simulink model "Feeder_1"  (Simulink 8.8)
settings: Solver=ode4  StartTime=0.0  StopTime=inf  FixedStep=Ts  RelTol=1e-3  EnableMultiTasking=on
PreLoadFcn:
  | Ts=125e-6;Core_Num = 0; np=1; nq=1; Vmin=.9;
PostLoadFcn:
  | Ts=125e-6;Core_Num = 0; np=1; nq=1; Vmin=.9;
InitFcn:
  | Ts=125e-6;Core_Num = 0; np=1; nq=1; Vmin=.9;
undefined symbols (not defined in the file or in its folder): another_event_name, DiscIntNeverNeededParam, I, j, Left, my_event_name, Right, type, V, X
libraries: powerlib x316, powerlib_meascontrol x227, simulink_extras x78, simulink x25, rtio_generic_c37_118 x22, ssn_lib x9, rtlab x6, powerlib_extras x3, artemis x1, rtio_opalrt_ml605ex1 x1, rtio_spectracom x1, rtio_generic_ethernet x1
(part 8 of 14)

== system Feeder_1/SS_PMU/Subsystem42/Subsystem ==
  In1 : Inport
  Bus Creator : BusCreator  Inputs=3
  Selector1 : Selector  InputPortWidth=14  IndexOptions=Index vector (dialog)  Indices=[13]  OutputSizes=1
  Selector2 : Selector  InputPortWidth=14  IndexOptions=Index vector (dialog)  Indices=[14]  OutputSizes=1
  Selector5 : Selector  InputPortWidth=14  IndexOptions=Index vector (dialog)  Indices=[1 2 3 4 5 6 7 8 9 10 11 12]  OutputSizes=1
  Out1 : Outport
  wires:
  In1/1 -> Selector5/1, Selector2/1, Selector1/1
  Selector5/1 -> Bus Creator/1  "Measurements"
  Bus Creator/1 -> Out1/1
  Selector1/1 -> Bus Creator/2  "FREQ"
  Selector2/1 -> Bus Creator/3  "FROC"

== system Feeder_1/SS_PMU/Subsystem43/Subsystem ==
  In1 : Inport
  Bus Creator : BusCreator  Inputs=3
  Selector1 : Selector  InputPortWidth=14  IndexOptions=Index vector (dialog)  Indices=[13]  OutputSizes=1
  Selector2 : Selector  InputPortWidth=14  IndexOptions=Index vector (dialog)  Indices=[14]  OutputSizes=1
  Selector5 : Selector  InputPortWidth=14  IndexOptions=Index vector (dialog)  Indices=[1 2 3 4 5 6 7 8 9 10 11 12]  OutputSizes=1
  Out1 : Outport
  wires:
  In1/1 -> Selector5/1, Selector2/1, Selector1/1
  Selector5/1 -> Bus Creator/1  "Measurements"
  Bus Creator/1 -> Out1/1
  Selector1/1 -> Bus Creator/2  "FREQ"
  Selector2/1 -> Bus Creator/3  "FROC"

== system Feeder_1/SS_PMU/Subsystem44/Subsystem ==
  In1 : Inport
  Bus Creator : BusCreator  Inputs=3
  Selector1 : Selector  InputPortWidth=14  IndexOptions=Index vector (dialog)  Indices=[13]  OutputSizes=1
  Selector2 : Selector  InputPortWidth=14  IndexOptions=Index vector (dialog)  Indices=[14]  OutputSizes=1
  Selector5 : Selector  InputPortWidth=14  IndexOptions=Index vector (dialog)  Indices=[1 2 3 4 5 6 7 8 9 10 11 12]  OutputSizes=1
  Out1 : Outport
  wires:
  In1/1 -> Selector5/1, Selector2/1, Selector1/1
  Selector5/1 -> Bus Creator/1  "Measurements"
  Bus Creator/1 -> Out1/1
  Selector1/1 -> Bus Creator/2  "FREQ"
  Selector2/1 -> Bus Creator/3  "FROC"

== system Feeder_1/SS_PMU/Subsystem5/Subsystem ==
  Measurements1 : Inport
  Demux7 : Demux  Outputs=2
  Subsystem1 : Subsystem
  Phasors_Vabc : Outport
  Phasors_Iabc : Outport  Port=2
  Phasor_Freq : Outport  Port=3
  Phasor_DTFreq : Outport  Port=4
  wires:
  Measurements1/1 -> Subsystem1/1(Measurements)
  Subsystem1/2(Phasors_Freq) -> Phasor_Freq/1
  Subsystem1/3(Phasors_DTFreq) -> Phasor_DTFreq/1
  Demux7/2 -> Phasors_Iabc/1
  Demux7/1 -> Phasors_Vabc/1
  Subsystem1/1(Phasors_abc) -> Demux7/1

== system Feeder_1/SS_PMU/Subsystem6/Subsystem ==
  Measurements1 : Inport
  Demux7 : Demux  Outputs=2
  Subsystem1 : Subsystem
  Phasors_Vabc : Outport
  Phasors_Iabc : Outport  Port=2
  Phasor_Freq : Outport  Port=3
  Phasor_DTFreq : Outport  Port=4
  wires:
  Measurements1/1 -> Subsystem1/1(Measurements)
  Subsystem1/2(Phasors_Freq) -> Phasor_Freq/1
  Subsystem1/3(Phasors_DTFreq) -> Phasor_DTFreq/1
  Demux7/2 -> Phasors_Iabc/1
  Demux7/1 -> Phasors_Vabc/1
  Subsystem1/1(Phasors_abc) -> Demux7/1

== system Feeder_1/SS_PMU/Subsystem7/Subsystem ==
  Measurements1 : Inport
  Demux7 : Demux  Outputs=2
  Subsystem1 : Subsystem
  Phasors_Vabc : Outport
  Phasors_Iabc : Outport  Port=2
  Phasor_Freq : Outport  Port=3
  Phasor_DTFreq : Outport  Port=4
  wires:
  Measurements1/1 -> Subsystem1/1(Measurements)
  Subsystem1/2(Phasors_Freq) -> Phasor_Freq/1
  Subsystem1/3(Phasors_DTFreq) -> Phasor_DTFreq/1
  Demux7/2 -> Phasors_Iabc/1
  Demux7/1 -> Phasors_Vabc/1
  Subsystem1/1(Phasors_abc) -> Demux7/1

== system Feeder_1/SS_PMU/Subsystem8/Subsystem ==
  Measurements1 : Inport
  Demux7 : Demux  Outputs=2
  Subsystem1 : Subsystem
  Phasors_Vabc : Outport
  Phasors_Iabc : Outport  Port=2
  Phasor_Freq : Outport  Port=3
  Phasor_DTFreq : Outport  Port=4
  wires:
  Measurements1/1 -> Subsystem1/1(Measurements)
  Subsystem1/2(Phasors_Freq) -> Phasor_Freq/1
  Subsystem1/3(Phasors_DTFreq) -> Phasor_DTFreq/1
  Demux7/2 -> Phasors_Iabc/1
  Demux7/1 -> Phasors_Vabc/1
  Subsystem1/1(Phasors_abc) -> Demux7/1

== system Feeder_1/SS_PMU/Subsystem9/Subsystem ==
  Measurements1 : Inport
  Demux7 : Demux  Outputs=2
  Subsystem1 : Subsystem
  Phasors_Vabc : Outport
  Phasors_Iabc : Outport  Port=2
  Phasor_Freq : Outport  Port=3
  Phasor_DTFreq : Outport  Port=4
  wires:
  Measurements1/1 -> Subsystem1/1(Measurements)
  Subsystem1/2(Phasors_Freq) -> Phasor_Freq/1
  Subsystem1/3(Phasors_DTFreq) -> Phasor_DTFreq/1
  Demux7/2 -> Phasors_Iabc/1
  Demux7/1 -> Phasors_Vabc/1
  Subsystem1/1(Phasors_abc) -> Demux7/1

== system Feeder_1/SM_NG/Dynamic Load BCDC2/Single-Phase Dynamic Load1/model ==
  v : Inport
  PQ : Inport  Port=2
  Break  Alg. Loop1 : Subsystem
  Complex to Magnitude-Angle : ComplexToMagnitudeAngle
  Complex to Real-Imag1 : ComplexToRealImag
  Constant : Constant
  Demux : Demux  Outputs=2
  Divide : Product  Inputs=**
  Gain : Gain  Gain=1.0114
  IC1 : InitialCondition
  IC2 : InitialCondition
  Magnitude-Angle to Complex : MagnitudeAngleToComplex
  PLL : Subsystem  mask{freq=fnom}
      mask prompts: freq "Initial frequency (Hz)"
  Positive Sequence  current : Subsystem
  RMS1 : powerlib_meascontrol/Measurements/RMS  TrueRMS=on  Freq=fnom  RMSInit=1  Ts=0
  Real-Imag to Complex : RealImagToComplex
  Real-Imag to Complex1 : RealImagToComplex
  Sum : Sum
  Transfer Fcn1 : TransferFcn  Numerator=[1 290.1]  Denominator=[1 298.8]
  Trigonometric Function1 : Trigonometry
  V> pu : Gain  Gain=1/Vbase/sqrt(3)  SaturateOnIntegerOverflow=on  OutDataTypeStr=Inherit: Same as input  ParamDataTypeStr=Inherit: Same as input
  V> pu1 : Gain  Gain=sqrt(2)  SaturateOnIntegerOverflow=on  OutDataTypeStr=Inherit: Same as input  ParamDataTypeStr=Inherit: Same as input
  i : Outport
  wires:
  V> pu/1 -> PLL/1(v (pu)), V> pu1/1
  Real-Imag to Complex/1 -> Positive Sequence  current/1(V1(pu))
  PQ/1 -> Demux/1
  Demux/1 -> Real-Imag to Complex1/1
  Demux/2 -> Real-Imag to Complex1/2
  Real-Imag to Complex1/1 -> Positive Sequence  current/2(S_ext)
  Complex to Real-Imag1/1 -> Real-Imag to Complex/1
  Complex to Real-Imag1/2 -> Real-Imag to Complex/2
  Magnitude-Angle to Complex/1 -> Complex to Real-Imag1/1
  Constant/1 -> PLL/2(freq (pu))
  PLL/1(alpha (rad)) -> Magnitude-Angle to Complex/2
  Complex to Magnitude-Angle/2 -> Sum/2
  PLL/2(wt) -> Sum/1
  Sum/1 -> Trigonometric Function1/1
  Trigonometric Function1/1 -> Divide/2
  Complex to Magnitude-Angle/1 -> Divide/1
  RMS1/1 -> IC1/1
  V> pu1/1 -> RMS1/1
  v/1 -> IC2/1
  Positive Sequence  current/1(I1(A)) -> Break  Alg. Loop1/1(In)
  Break  Alg. Loop1/1(Out) -> Complex to Magnitude-Angle/1
  IC1/1 -> Magnitude-Angle to Complex/1
  IC2/1 -> V> pu/1
  Transfer Fcn1/1 -> Gain/1
  Gain/1 -> i/1
  Divide/1 -> Transfer Fcn1/1

== system Feeder_1/SM_NG/Dynamic Load BCDC2/Single-Phase Dynamic Load2/model ==
  v : Inport
  PQ : Inport  Port=2
  Break  Alg. Loop1 : Subsystem
  Complex to Magnitude-Angle : ComplexToMagnitudeAngle
  Complex to Real-Imag1 : ComplexToRealImag
  Constant : Constant
  Demux : Demux  Outputs=2
  Divide : Product  Inputs=**
  Gain : Gain  Gain=1.0114
  IC1 : InitialCondition
  IC2 : InitialCondition
  Magnitude-Angle to Complex : MagnitudeAngleToComplex
  PLL : Subsystem  mask{freq=fnom}
      mask prompts: freq "Initial frequency (Hz)"
  Positive Sequence  current : Subsystem
  RMS1 : powerlib_meascontrol/Measurements/RMS  TrueRMS=on  Freq=fnom  RMSInit=1  Ts=0
  Real-Imag to Complex : RealImagToComplex
  Real-Imag to Complex1 : RealImagToComplex
  Sum : Sum
  Transfer Fcn1 : TransferFcn  Numerator=[1 290.1]  Denominator=[1 298.8]
  Trigonometric Function1 : Trigonometry
  V> pu : Gain  Gain=1/Vbase/sqrt(3)  SaturateOnIntegerOverflow=on  OutDataTypeStr=Inherit: Same as input  ParamDataTypeStr=Inherit: Same as input
  V> pu1 : Gain  Gain=sqrt(2)  SaturateOnIntegerOverflow=on  OutDataTypeStr=Inherit: Same as input  ParamDataTypeStr=Inherit: Same as input
  i : Outport
  wires:
  V> pu/1 -> PLL/1(v (pu)), V> pu1/1
  Real-Imag to Complex/1 -> Positive Sequence  current/1(V1(pu))
  PQ/1 -> Demux/1
  Demux/1 -> Real-Imag to Complex1/1
  Demux/2 -> Real-Imag to Complex1/2
  Real-Imag to Complex1/1 -> Positive Sequence  current/2(S_ext)
  Complex to Real-Imag1/1 -> Real-Imag to Complex/1
  Complex to Real-Imag1/2 -> Real-Imag to Complex/2
  Magnitude-Angle to Complex/1 -> Complex to Real-Imag1/1
  Constant/1 -> PLL/2(freq (pu))
  PLL/1(alpha (rad)) -> Magnitude-Angle to Complex/2
  Complex to Magnitude-Angle/2 -> Sum/2
  PLL/2(wt) -> Sum/1
  Sum/1 -> Trigonometric Function1/1
  Trigonometric Function1/1 -> Divide/2
  Complex to Magnitude-Angle/1 -> Divide/1
  RMS1/1 -> IC1/1
  V> pu1/1 -> RMS1/1
  v/1 -> IC2/1
  Positive Sequence  current/1(I1(A)) -> Break  Alg. Loop1/1(In)
  Break  Alg. Loop1/1(Out) -> Complex to Magnitude-Angle/1
  IC1/1 -> Magnitude-Angle to Complex/1
  IC2/1 -> V> pu/1
  Transfer Fcn1/1 -> Gain/1
  Gain/1 -> i/1
  Divide/1 -> Transfer Fcn1/1

== system Feeder_1/SM_NG/Dynamic Load BCDC2/Single-Phase Dynamic Load9/model ==
  v : Inport
  PQ : Inport  Port=2
  Break  Alg. Loop1 : Subsystem
  Complex to Magnitude-Angle : ComplexToMagnitudeAngle
  Complex to Real-Imag1 : ComplexToRealImag
  Constant : Constant
  Demux : Demux  Outputs=2
  Divide : Product  Inputs=**
  Gain : Gain  Gain=1.0114
  IC1 : InitialCondition
  IC2 : InitialCondition
  Magnitude-Angle to Complex : MagnitudeAngleToComplex
  PLL : Subsystem  mask{freq=fnom}
      mask prompts: freq "Initial frequency (Hz)"
  Positive Sequence  current : Subsystem
  RMS1 : powerlib_meascontrol/Measurements/RMS  TrueRMS=on  Freq=fnom  RMSInit=1  Ts=0
  Real-Imag to Complex : RealImagToComplex
  Real-Imag to Complex1 : RealImagToComplex
  Sum : Sum
  Transfer Fcn1 : TransferFcn  Numerator=[1 290.1]  Denominator=[1 298.8]
  Trigonometric Function1 : Trigonometry
  V> pu : Gain  Gain=1/Vbase/sqrt(3)  SaturateOnIntegerOverflow=on  OutDataTypeStr=Inherit: Same as input  ParamDataTypeStr=Inherit: Same as input
  V> pu1 : Gain  Gain=sqrt(2)  SaturateOnIntegerOverflow=on  OutDataTypeStr=Inherit: Same as input  ParamDataTypeStr=Inherit: Same as input
  i : Outport
  wires:
  V> pu/1 -> PLL/1(v (pu)), V> pu1/1
  Real-Imag to Complex/1 -> Positive Sequence  current/1(V1(pu))
  PQ/1 -> Demux/1
  Demux/1 -> Real-Imag to Complex1/1
  Demux/2 -> Real-Imag to Complex1/2
  Real-Imag to Complex1/1 -> Positive Sequence  current/2(S_ext)
  Complex to Real-Imag1/1 -> Real-Imag to Complex/1
  Complex to Real-Imag1/2 -> Real-Imag to Complex/2
  Magnitude-Angle to Complex/1 -> Complex to Real-Imag1/1
  Constant/1 -> PLL/2(freq (pu))
  PLL/1(alpha (rad)) -> Magnitude-Angle to Complex/2
  Complex to Magnitude-Angle/2 -> Sum/2
  PLL/2(wt) -> Sum/1
  Sum/1 -> Trigonometric Function1/1
  Trigonometric Function1/1 -> Divide/2
  Complex to Magnitude-Angle/1 -> Divide/1
  RMS1/1 -> IC1/1
  V> pu1/1 -> RMS1/1
  v/1 -> IC2/1
  Positive Sequence  current/1(I1(A)) -> Break  Alg. Loop1/1(In)
  Break  Alg. Loop1/1(Out) -> Complex to Magnitude-Angle/1
  IC1/1 -> Magnitude-Angle to Complex/1
  IC2/1 -> V> pu/1
  Transfer Fcn1/1 -> Gain/1
  Gain/1 -> i/1
  Divide/1 -> Transfer Fcn1/1

== system Feeder_1/SM_NG/Dynamic Load BCDC3/Single-Phase Dynamic Load1/model ==
  v : Inport
  PQ : Inport  Port=2
  Break  Alg. Loop1 : Subsystem
  Complex to Magnitude-Angle : ComplexToMagnitudeAngle
  Complex to Real-Imag1 : ComplexToRealImag
  Constant : Constant
  Demux : Demux  Outputs=2
  Divide : Product  Inputs=**
  Gain : Gain  Gain=1.0114
  IC1 : InitialCondition
  IC2 : InitialCondition
  Magnitude-Angle to Complex : MagnitudeAngleToComplex
  PLL : Subsystem  mask{freq=fnom}
      mask prompts: freq "Initial frequency (Hz)"
  Positive Sequence  current : Subsystem
  RMS1 : powerlib_meascontrol/Measurements/RMS  TrueRMS=on  Freq=fnom  RMSInit=1  Ts=0
  Real-Imag to Complex : RealImagToComplex
  Real-Imag to Complex1 : RealImagToComplex
  Sum : Sum
  Transfer Fcn1 : TransferFcn  Numerator=[1 290.1]  Denominator=[1 298.8]
  Trigonometric Function1 : Trigonometry
  V> pu : Gain  Gain=1/Vbase/sqrt(3)  SaturateOnIntegerOverflow=on  OutDataTypeStr=Inherit: Same as input  ParamDataTypeStr=Inherit: Same as input
  V> pu1 : Gain  Gain=sqrt(2)  SaturateOnIntegerOverflow=on  OutDataTypeStr=Inherit: Same as input  ParamDataTypeStr=Inherit: Same as input
  i : Outport
  wires:
  V> pu/1 -> PLL/1(v (pu)), V> pu1/1
  Real-Imag to Complex/1 -> Positive Sequence  current/1(V1(pu))
  PQ/1 -> Demux/1
  Demux/1 -> Real-Imag to Complex1/1
  Demux/2 -> Real-Imag to Complex1/2
  Real-Imag to Complex1/1 -> Positive Sequence  current/2(S_ext)
  Complex to Real-Imag1/1 -> Real-Imag to Complex/1
  Complex to Real-Imag1/2 -> Real-Imag to Complex/2
  Magnitude-Angle to Complex/1 -> Complex to Real-Imag1/1
  Constant/1 -> PLL/2(freq (pu))
  PLL/1(alpha (rad)) -> Magnitude-Angle to Complex/2
  Complex to Magnitude-Angle/2 -> Sum/2
  PLL/2(wt) -> Sum/1
  Sum/1 -> Trigonometric Function1/1
  Trigonometric Function1/1 -> Divide/2
  Complex to Magnitude-Angle/1 -> Divide/1
  RMS1/1 -> IC1/1
  V> pu1/1 -> RMS1/1
  v/1 -> IC2/1
  Positive Sequence  current/1(I1(A)) -> Break  Alg. Loop1/1(In)
  Break  Alg. Loop1/1(Out) -> Complex to Magnitude-Angle/1
  IC1/1 -> Magnitude-Angle to Complex/1
  IC2/1 -> V> pu/1
  Transfer Fcn1/1 -> Gain/1
  Gain/1 -> i/1
  Divide/1 -> Transfer Fcn1/1

== system Feeder_1/SM_NG/Dynamic Load BCDC3/Single-Phase Dynamic Load2/model ==
  v : Inport
  PQ : Inport  Port=2
  Break  Alg. Loop1 : Subsystem
  Complex to Magnitude-Angle : ComplexToMagnitudeAngle
  Complex to Real-Imag1 : ComplexToRealImag
  Constant : Constant
  Demux : Demux  Outputs=2
  Divide : Product  Inputs=**
  Gain : Gain  Gain=1.0114
  IC1 : InitialCondition
  IC2 : InitialCondition
  Magnitude-Angle to Complex : MagnitudeAngleToComplex
  PLL : Subsystem  mask{freq=fnom}
      mask prompts: freq "Initial frequency (Hz)"
  Positive Sequence  current : Subsystem
  RMS1 : powerlib_meascontrol/Measurements/RMS  TrueRMS=on  Freq=fnom  RMSInit=1  Ts=0
  Real-Imag to Complex : RealImagToComplex
  Real-Imag to Complex1 : RealImagToComplex
  Sum : Sum
  Transfer Fcn1 : TransferFcn  Numerator=[1 290.1]  Denominator=[1 298.8]
  Trigonometric Function1 : Trigonometry
  V> pu : Gain  Gain=1/Vbase/sqrt(3)  SaturateOnIntegerOverflow=on  OutDataTypeStr=Inherit: Same as input  ParamDataTypeStr=Inherit: Same as input
  V> pu1 : Gain  Gain=sqrt(2)  SaturateOnIntegerOverflow=on  OutDataTypeStr=Inherit: Same as input  ParamDataTypeStr=Inherit: Same as input
  i : Outport
  wires:
  V> pu/1 -> PLL/1(v (pu)), V> pu1/1
  Real-Imag to Complex/1 -> Positive Sequence  current/1(V1(pu))
  PQ/1 -> Demux/1
  Demux/1 -> Real-Imag to Complex1/1
  Demux/2 -> Real-Imag to Complex1/2
  Real-Imag to Complex1/1 -> Positive Sequence  current/2(S_ext)
  Complex to Real-Imag1/1 -> Real-Imag to Complex/1
  Complex to Real-Imag1/2 -> Real-Imag to Complex/2
  Magnitude-Angle to Complex/1 -> Complex to Real-Imag1/1
  Constant/1 -> PLL/2(freq (pu))
  PLL/1(alpha (rad)) -> Magnitude-Angle to Complex/2
  Complex to Magnitude-Angle/2 -> Sum/2
  PLL/2(wt) -> Sum/1
  Sum/1 -> Trigonometric Function1/1
  Trigonometric Function1/1 -> Divide/2
  Complex to Magnitude-Angle/1 -> Divide/1
  RMS1/1 -> IC1/1
  V> pu1/1 -> RMS1/1
  v/1 -> IC2/1
  Positive Sequence  current/1(I1(A)) -> Break  Alg. Loop1/1(In)
  Break  Alg. Loop1/1(Out) -> Complex to Magnitude-Angle/1
  IC1/1 -> Magnitude-Angle to Complex/1
  IC2/1 -> V> pu/1
  Transfer Fcn1/1 -> Gain/1
  Gain/1 -> i/1
  Divide/1 -> Transfer Fcn1/1

== system Feeder_1/SM_NG/Dynamic Load BCDC3/Single-Phase Dynamic Load9/model ==
  v : Inport
  PQ : Inport  Port=2
  Break  Alg. Loop1 : Subsystem
  Complex to Magnitude-Angle : ComplexToMagnitudeAngle
  Complex to Real-Imag1 : ComplexToRealImag
  Constant : Constant
  Demux : Demux  Outputs=2
  Divide : Product  Inputs=**
  Gain : Gain  Gain=1.0114
  IC1 : InitialCondition
  IC2 : InitialCondition
  Magnitude-Angle to Complex : MagnitudeAngleToComplex
  PLL : Subsystem  mask{freq=fnom}
      mask prompts: freq "Initial frequency (Hz)"
  Positive Sequence  current : Subsystem
  RMS1 : powerlib_meascontrol/Measurements/RMS  TrueRMS=on  Freq=fnom  RMSInit=1  Ts=0
  Real-Imag to Complex : RealImagToComplex
  Real-Imag to Complex1 : RealImagToComplex
  Sum : Sum
  Transfer Fcn1 : TransferFcn  Numerator=[1 290.1]  Denominator=[1 298.8]
  Trigonometric Function1 : Trigonometry
  V> pu : Gain  Gain=1/Vbase/sqrt(3)  SaturateOnIntegerOverflow=on  OutDataTypeStr=Inherit: Same as input  ParamDataTypeStr=Inherit: Same as input
  V> pu1 : Gain  Gain=sqrt(2)  SaturateOnIntegerOverflow=on  OutDataTypeStr=Inherit: Same as input  ParamDataTypeStr=Inherit: Same as input
  i : Outport
  wires:
  V> pu/1 -> PLL/1(v (pu)), V> pu1/1
  Real-Imag to Complex/1 -> Positive Sequence  current/1(V1(pu))
  PQ/1 -> Demux/1
  Demux/1 -> Real-Imag to Complex1/1
  Demux/2 -> Real-Imag to Complex1/2
  Real-Imag to Complex1/1 -> Positive Sequence  current/2(S_ext)
  Complex to Real-Imag1/1 -> Real-Imag to Complex/1
  Complex to Real-Imag1/2 -> Real-Imag to Complex/2
  Magnitude-Angle to Complex/1 -> Complex to Real-Imag1/1
  Constant/1 -> PLL/2(freq (pu))
  PLL/1(alpha (rad)) -> Magnitude-Angle to Complex/2
  Complex to Magnitude-Angle/2 -> Sum/2
  PLL/2(wt) -> Sum/1
  Sum/1 -> Trigonometric Function1/1
  Trigonometric Function1/1 -> Divide/2
  Complex to Magnitude-Angle/1 -> Divide/1
  RMS1/1 -> IC1/1
  V> pu1/1 -> RMS1/1
  v/1 -> IC2/1
  Positive Sequence  current/1(I1(A)) -> Break  Alg. Loop1/1(In)
  Break  Alg. Loop1/1(Out) -> Complex to Magnitude-Angle/1
  IC1/1 -> Magnitude-Angle to Complex/1
  IC2/1 -> V> pu/1
  Transfer Fcn1/1 -> Gain/1
  Gain/1 -> i/1
  Divide/1 -> Transfer Fcn1/1

== system Feeder_1/SM_NG/Dynamic Load BCDC4/Single-Phase Dynamic Load1/model ==
  v : Inport
  PQ : Inport  Port=2
  Break  Alg. Loop1 : Subsystem
  Complex to Magnitude-Angle : ComplexToMagnitudeAngle
  Complex to Real-Imag1 : ComplexToRealImag
  Constant : Constant
  Demux : Demux  Outputs=2
  Divide : Product  Inputs=**
  Gain : Gain  Gain=1.0114
  IC1 : InitialCondition
  IC2 : InitialCondition
  Magnitude-Angle to Complex : MagnitudeAngleToComplex
  PLL : Subsystem  mask{freq=fnom}
      mask prompts: freq "Initial frequency (Hz)"
  Positive Sequence  current : Subsystem
  RMS1 : powerlib_meascontrol/Measurements/RMS  TrueRMS=on  Freq=fnom  RMSInit=1  Ts=0
  Real-Imag to Complex : RealImagToComplex
  Real-Imag to Complex1 : RealImagToComplex
  Sum : Sum
  Transfer Fcn1 : TransferFcn  Numerator=[1 290.1]  Denominator=[1 298.8]
  Trigonometric Function1 : Trigonometry
  V> pu : Gain  Gain=1/Vbase/sqrt(3)  SaturateOnIntegerOverflow=on  OutDataTypeStr=Inherit: Same as input  ParamDataTypeStr=Inherit: Same as input
  V> pu1 : Gain  Gain=sqrt(2)  SaturateOnIntegerOverflow=on  OutDataTypeStr=Inherit: Same as input  ParamDataTypeStr=Inherit: Same as input
  i : Outport
  wires:
  V> pu/1 -> PLL/1(v (pu)), V> pu1/1
  Real-Imag to Complex/1 -> Positive Sequence  current/1(V1(pu))
  PQ/1 -> Demux/1
  Demux/1 -> Real-Imag to Complex1/1
  Demux/2 -> Real-Imag to Complex1/2
  Real-Imag to Complex1/1 -> Positive Sequence  current/2(S_ext)
  Complex to Real-Imag1/1 -> Real-Imag to Complex/1
  Complex to Real-Imag1/2 -> Real-Imag to Complex/2
  Magnitude-Angle to Complex/1 -> Complex to Real-Imag1/1
  Constant/1 -> PLL/2(freq (pu))
  PLL/1(alpha (rad)) -> Magnitude-Angle to Complex/2
  Complex to Magnitude-Angle/2 -> Sum/2
  PLL/2(wt) -> Sum/1
  Sum/1 -> Trigonometric Function1/1
  Trigonometric Function1/1 -> Divide/2
  Complex to Magnitude-Angle/1 -> Divide/1
  RMS1/1 -> IC1/1
  V> pu1/1 -> RMS1/1
  v/1 -> IC2/1
  Positive Sequence  current/1(I1(A)) -> Break  Alg. Loop1/1(In)
  Break  Alg. Loop1/1(Out) -> Complex to Magnitude-Angle/1
  IC1/1 -> Magnitude-Angle to Complex/1
  IC2/1 -> V> pu/1
  Transfer Fcn1/1 -> Gain/1
  Gain/1 -> i/1
  Divide/1 -> Transfer Fcn1/1

== system Feeder_1/SM_NG/Dynamic Load BCDC4/Single-Phase Dynamic Load2/model ==
  v : Inport
  PQ : Inport  Port=2
  Break  Alg. Loop1 : Subsystem
  Complex to Magnitude-Angle : ComplexToMagnitudeAngle
  Complex to Real-Imag1 : ComplexToRealImag
  Constant : Constant
  Demux : Demux  Outputs=2
  Divide : Product  Inputs=**
  Gain : Gain  Gain=1.0114
  IC1 : InitialCondition
  IC2 : InitialCondition
  Magnitude-Angle to Complex : MagnitudeAngleToComplex
  PLL : Subsystem  mask{freq=fnom}
      mask prompts: freq "Initial frequency (Hz)"
  Positive Sequence  current : Subsystem
  RMS1 : powerlib_meascontrol/Measurements/RMS  TrueRMS=on  Freq=fnom  RMSInit=1  Ts=0
  Real-Imag to Complex : RealImagToComplex
  Real-Imag to Complex1 : RealImagToComplex
  Sum : Sum
  Transfer Fcn1 : TransferFcn  Numerator=[1 290.1]  Denominator=[1 298.8]
  Trigonometric Function1 : Trigonometry
  V> pu : Gain  Gain=1/Vbase/sqrt(3)  SaturateOnIntegerOverflow=on  OutDataTypeStr=Inherit: Same as input  ParamDataTypeStr=Inherit: Same as input
  V> pu1 : Gain  Gain=sqrt(2)  SaturateOnIntegerOverflow=on  OutDataTypeStr=Inherit: Same as input  ParamDataTypeStr=Inherit: Same as input
  i : Outport
  wires:
  V> pu/1 -> PLL/1(v (pu)), V> pu1/1
  Real-Imag to Complex/1 -> Positive Sequence  current/1(V1(pu))
  PQ/1 -> Demux/1
  Demux/1 -> Real-Imag to Complex1/1
  Demux/2 -> Real-Imag to Complex1/2
  Real-Imag to Complex1/1 -> Positive Sequence  current/2(S_ext)
  Complex to Real-Imag1/1 -> Real-Imag to Complex/1
  Complex to Real-Imag1/2 -> Real-Imag to Complex/2
  Magnitude-Angle to Complex/1 -> Complex to Real-Imag1/1
  Constant/1 -> PLL/2(freq (pu))
  PLL/1(alpha (rad)) -> Magnitude-Angle to Complex/2
  Complex to Magnitude-Angle/2 -> Sum/2
  PLL/2(wt) -> Sum/1
  Sum/1 -> Trigonometric Function1/1
  Trigonometric Function1/1 -> Divide/2
  Complex to Magnitude-Angle/1 -> Divide/1
  RMS1/1 -> IC1/1
  V> pu1/1 -> RMS1/1
  v/1 -> IC2/1
  Positive Sequence  current/1(I1(A)) -> Break  Alg. Loop1/1(In)
  Break  Alg. Loop1/1(Out) -> Complex to Magnitude-Angle/1
  IC1/1 -> Magnitude-Angle to Complex/1
  IC2/1 -> V> pu/1
  Transfer Fcn1/1 -> Gain/1
  Gain/1 -> i/1
  Divide/1 -> Transfer Fcn1/1

== system Feeder_1/SM_NG/Dynamic Load BCDC4/Single-Phase Dynamic Load9/model ==
  v : Inport
  PQ : Inport  Port=2
  Break  Alg. Loop1 : Subsystem
  Complex to Magnitude-Angle : ComplexToMagnitudeAngle
  Complex to Real-Imag1 : ComplexToRealImag
  Constant : Constant
  Demux : Demux  Outputs=2
  Divide : Product  Inputs=**
  Gain : Gain  Gain=1.0114
  IC1 : InitialCondition
  IC2 : InitialCondition
  Magnitude-Angle to Complex : MagnitudeAngleToComplex
  PLL : Subsystem  mask{freq=fnom}
      mask prompts: freq "Initial frequency (Hz)"
  Positive Sequence  current : Subsystem
  RMS1 : powerlib_meascontrol/Measurements/RMS  TrueRMS=on  Freq=fnom  RMSInit=1  Ts=0
  Real-Imag to Complex : RealImagToComplex
  Real-Imag to Complex1 : RealImagToComplex
  Sum : Sum
  Transfer Fcn1 : TransferFcn  Numerator=[1 290.1]  Denominator=[1 298.8]
  Trigonometric Function1 : Trigonometry
  V> pu : Gain  Gain=1/Vbase/sqrt(3)  SaturateOnIntegerOverflow=on  OutDataTypeStr=Inherit: Same as input  ParamDataTypeStr=Inherit: Same as input
  V> pu1 : Gain  Gain=sqrt(2)  SaturateOnIntegerOverflow=on  OutDataTypeStr=Inherit: Same as input  ParamDataTypeStr=Inherit: Same as input
  i : Outport
  wires:
  V> pu/1 -> PLL/1(v (pu)), V> pu1/1
  Real-Imag to Complex/1 -> Positive Sequence  current/1(V1(pu))
  PQ/1 -> Demux/1
  Demux/1 -> Real-Imag to Complex1/1
  Demux/2 -> Real-Imag to Complex1/2
  Real-Imag to Complex1/1 -> Positive Sequence  current/2(S_ext)
  Complex to Real-Imag1/1 -> Real-Imag to Complex/1
  Complex to Real-Imag1/2 -> Real-Imag to Complex/2
  Magnitude-Angle to Complex/1 -> Complex to Real-Imag1/1
  Constant/1 -> PLL/2(freq (pu))
  PLL/1(alpha (rad)) -> Magnitude-Angle to Complex/2
  Complex to Magnitude-Angle/2 -> Sum/2
  PLL/2(wt) -> Sum/1
  Sum/1 -> Trigonometric Function1/1
  Trigonometric Function1/1 -> Divide/2
  Complex to Magnitude-Angle/1 -> Divide/1
  RMS1/1 -> IC1/1
  V> pu1/1 -> RMS1/1
  v/1 -> IC2/1
  Positive Sequence  current/1(I1(A)) -> Break  Alg. Loop1/1(In)
  Break  Alg. Loop1/1(Out) -> Complex to Magnitude-Angle/1
  IC1/1 -> Magnitude-Angle to Complex/1
  IC2/1 -> V> pu/1
  Transfer Fcn1/1 -> Gain/1
  Gain/1 -> i/1
  Divide/1 -> Transfer Fcn1/1

== system Feeder_1/SM_NG/Single-Phase Dynamic Load30/model/Break  Alg. Loop1 ==
  In : Inport
  Complex to Real-Imag : ComplexToRealImag
  Real-Imag to Complex : RealImagToComplex
  imag : simulink_extras/Additional Linear/Transfer Fcn (with initial outputs)  N=[1]  D="[100e-6  1]"  Y0=imag(I1_init*exp(-j*Pha_V0*pi/180))  U0=imag(I1_init*exp(-j*Pha_V0*pi/180))
  real : simulink_extras/Additional Linear/Transfer Fcn (with initial outputs)  N=[1]  D="[100e-6  1]"  Y0=real(I1_init*exp(-j*Pha_V0*pi/180))  U0=real(I1_init*exp(-j*Pha_V0*pi/180))
  Out : Outport
  wires:
  Complex to Real-Imag/2 -> imag/1
  Complex to Real-Imag/1 -> real/1
  Real-Imag to Complex/1 -> Out/1
  In/1 -> Complex to Real-Imag/1
  imag/1 -> Real-Imag to Complex/2
  real/1 -> Real-Imag to Complex/1

== system Feeder_1/SM_NG/Single-Phase Dynamic Load30/model/PLL ==
  v (pu) : Inport
  freq (pu) : Inport  Port=2
  Gain : Gain  Gain=2*pi
  Gain1 : Gain  Gain=500
  Gain2 : Gain  Gain=freq
  IC : InitialCondition
  Integrator : Integrator
  Integrator1 : Integrator
  Product : Product  Inputs=**  RndMeth=Zero
  Sum1 : Sum  SaturateOnIntegerOverflow=on  InputSameDT=on  OutDataTypeStr=Inherit: Same as first input
  Trigonometric Function : Trigonometry  Operator=cos
  adaptive filter : Subsystem
  adaptive mean : Subsystem
  alpha (rad) : Outport
  wt : Outport  Port=2
  wires:
  freq (pu)/1 -> Gain2/1
  Gain2/1 -> adaptive filter/2(freq (Hz)), adaptive mean/2(freq (Hz)), Gain/1
  Trigonometric Function/1 -> Product/2
  adaptive mean/1(y) -> alpha (rad)/1
  Integrator1/1 -> Gain1/1
  Gain1/1 -> Sum1/1, adaptive mean/1(u)
  Sum1/1 -> Trigonometric Function/1
  Integrator/1 -> Sum1/2, wt/1
  Gain/1 -> Integrator/1
  adaptive filter/1(y) -> Integrator1/1
  Product/1 -> adaptive filter/1(u)
  v (pu)/1 -> IC/1
  IC/1 -> Product/1

== system Feeder_1/SM_NG/Single-Phase Dynamic Load30/model/Positive Sequence  current ==
  note: I1= (S/V1)'
  V1(pu) : Inport
  S_ext : Inport  Port=2
  Conj1 : Math  Operator=conj  SaturateOnIntegerOverflow=on
  Product : Product  Inputs=/*  SaturateOnIntegerOverflow=on  InputSameDT=on  OutDataTypeStr=Inherit: Same as first input
  pu>V : Gain  Gain=Vnom/sqrt(2)  SaturateOnIntegerOverflow=on  OutDataTypeStr=Inherit: Same as input  ParamDataTypeStr=Inherit: Same as input
  I1(A) : Outport
  wires:
  V1(pu)/1 -> pu>V/1
  Product/1 -> Conj1/1
  Conj1/1 -> I1(A)/1
  S_ext/1 -> Product/2
  pu>V/1 -> Product/1

== system Feeder_1/SM_NG/Single-Phase Dynamic Load32/model/Break  Alg. Loop1 ==
  In : Inport
  Complex to Real-Imag : ComplexToRealImag
  Real-Imag to Complex : RealImagToComplex
  imag : simulink_extras/Additional Linear/Transfer Fcn (with initial outputs)  N=[1]  D="[100e-6  1]"  Y0=imag(I1_init*exp(-j*Pha_V0*pi/180))  U0=imag(I1_init*exp(-j*Pha_V0*pi/180))
  real : simulink_extras/Additional Linear/Transfer Fcn (with initial outputs)  N=[1]  D="[100e-6  1]"  Y0=real(I1_init*exp(-j*Pha_V0*pi/180))  U0=real(I1_init*exp(-j*Pha_V0*pi/180))
  Out : Outport
  wires:
  Complex to Real-Imag/2 -> imag/1
  Complex to Real-Imag/1 -> real/1
  Real-Imag to Complex/1 -> Out/1
  In/1 -> Complex to Real-Imag/1
  imag/1 -> Real-Imag to Complex/2
  real/1 -> Real-Imag to Complex/1

== system Feeder_1/SM_NG/Single-Phase Dynamic Load32/model/PLL ==
  v (pu) : Inport
  freq (pu) : Inport  Port=2
  Gain : Gain  Gain=2*pi
  Gain1 : Gain  Gain=500
  Gain2 : Gain  Gain=freq
  IC : InitialCondition
  Integrator : Integrator
  Integrator1 : Integrator
  Product : Product  Inputs=**  RndMeth=Zero
  Sum1 : Sum  SaturateOnIntegerOverflow=on  InputSameDT=on  OutDataTypeStr=Inherit: Same as first input
  Trigonometric Function : Trigonometry  Operator=cos
  adaptive filter : Subsystem
  adaptive mean : Subsystem
  alpha (rad) : Outport
  wt : Outport  Port=2
  wires:
  freq (pu)/1 -> Gain2/1
  Gain2/1 -> adaptive filter/2(freq (Hz)), adaptive mean/2(freq (Hz)), Gain/1
  Trigonometric Function/1 -> Product/2
  adaptive mean/1(y) -> alpha (rad)/1
  Integrator1/1 -> Gain1/1
  Gain1/1 -> Sum1/1, adaptive mean/1(u)
  Sum1/1 -> Trigonometric Function/1
  Integrator/1 -> Sum1/2, wt/1
  Gain/1 -> Integrator/1
  adaptive filter/1(y) -> Integrator1/1
  Product/1 -> adaptive filter/1(u)
  v (pu)/1 -> IC/1
  IC/1 -> Product/1

== system Feeder_1/SM_NG/Single-Phase Dynamic Load32/model/Positive Sequence  current ==
  note: I1= (S/V1)'
  V1(pu) : Inport
  S_ext : Inport  Port=2
  Conj1 : Math  Operator=conj  SaturateOnIntegerOverflow=on
  Product : Product  Inputs=/*  SaturateOnIntegerOverflow=on  InputSameDT=on  OutDataTypeStr=Inherit: Same as first input
  pu>V : Gain  Gain=Vnom/sqrt(2)  SaturateOnIntegerOverflow=on  OutDataTypeStr=Inherit: Same as input  ParamDataTypeStr=Inherit: Same as input
  I1(A) : Outport
  wires:
  V1(pu)/1 -> pu>V/1
  Product/1 -> Conj1/1
  Conj1/1 -> I1(A)/1
  S_ext/1 -> Product/2
  pu>V/1 -> Product/1

== system Feeder_1/SM_NG/Single-Phase Dynamic Load33/model/Break  Alg. Loop1 ==
  In : Inport
  Complex to Real-Imag : ComplexToRealImag
  Real-Imag to Complex : RealImagToComplex
  imag : simulink_extras/Additional Linear/Transfer Fcn (with initial outputs)  N=[1]  D="[100e-6  1]"  Y0=imag(I1_init*exp(-j*Pha_V0*pi/180))  U0=imag(I1_init*exp(-j*Pha_V0*pi/180))
  real : simulink_extras/Additional Linear/Transfer Fcn (with initial outputs)  N=[1]  D="[100e-6  1]"  Y0=real(I1_init*exp(-j*Pha_V0*pi/180))  U0=real(I1_init*exp(-j*Pha_V0*pi/180))
  Out : Outport
  wires:
  Complex to Real-Imag/2 -> imag/1
  Complex to Real-Imag/1 -> real/1
  Real-Imag to Complex/1 -> Out/1
  In/1 -> Complex to Real-Imag/1
  imag/1 -> Real-Imag to Complex/2
  real/1 -> Real-Imag to Complex/1

== system Feeder_1/SM_NG/Single-Phase Dynamic Load33/model/PLL ==
  v (pu) : Inport
  freq (pu) : Inport  Port=2
  Gain : Gain  Gain=2*pi
  Gain1 : Gain  Gain=500
  Gain2 : Gain  Gain=freq
  IC : InitialCondition
  Integrator : Integrator
  Integrator1 : Integrator
  Product : Product  Inputs=**  RndMeth=Zero
  Sum1 : Sum  SaturateOnIntegerOverflow=on  InputSameDT=on  OutDataTypeStr=Inherit: Same as first input
  Trigonometric Function : Trigonometry  Operator=cos
  adaptive filter : Subsystem
  adaptive mean : Subsystem
  alpha (rad) : Outport
  wt : Outport  Port=2
  wires:
  freq (pu)/1 -> Gain2/1
  Gain2/1 -> adaptive filter/2(freq (Hz)), adaptive mean/2(freq (Hz)), Gain/1
  Trigonometric Function/1 -> Product/2
  adaptive mean/1(y) -> alpha (rad)/1
  Integrator1/1 -> Gain1/1
  Gain1/1 -> Sum1/1, adaptive mean/1(u)
  Sum1/1 -> Trigonometric Function/1
  Integrator/1 -> Sum1/2, wt/1
  Gain/1 -> Integrator/1
  adaptive filter/1(y) -> Integrator1/1
  Product/1 -> adaptive filter/1(u)
  v (pu)/1 -> IC/1
  IC/1 -> Product/1

== system Feeder_1/SM_NG/Single-Phase Dynamic Load33/model/Positive Sequence  current ==
  note: I1= (S/V1)'
  V1(pu) : Inport
  S_ext : Inport  Port=2
  Conj1 : Math  Operator=conj  SaturateOnIntegerOverflow=on
  Product : Product  Inputs=/*  SaturateOnIntegerOverflow=on  InputSameDT=on  OutDataTypeStr=Inherit: Same as first input
  pu>V : Gain  Gain=Vnom/sqrt(2)  SaturateOnIntegerOverflow=on  OutDataTypeStr=Inherit: Same as input  ParamDataTypeStr=Inherit: Same as input
  I1(A) : Outport
  wires:
  V1(pu)/1 -> pu>V/1
  Product/1 -> Conj1/1
  Conj1/1 -> I1(A)/1
  S_ext/1 -> Product/2
  pu>V/1 -> Product/1

== system Feeder_1/SM_NG/Single-Phase Dynamic Load34/model/Break  Alg. Loop1 ==
  In : Inport
  Complex to Real-Imag : ComplexToRealImag
  Real-Imag to Complex : RealImagToComplex
  imag : simulink_extras/Additional Linear/Transfer Fcn (with initial outputs)  N=[1]  D="[100e-6  1]"  Y0=imag(I1_init*exp(-j*Pha_V0*pi/180))  U0=imag(I1_init*exp(-j*Pha_V0*pi/180))
  real : simulink_extras/Additional Linear/Transfer Fcn (with initial outputs)  N=[1]  D="[100e-6  1]"  Y0=real(I1_init*exp(-j*Pha_V0*pi/180))  U0=real(I1_init*exp(-j*Pha_V0*pi/180))
  Out : Outport
  wires:
  Complex to Real-Imag/2 -> imag/1
  Complex to Real-Imag/1 -> real/1
  Real-Imag to Complex/1 -> Out/1
  In/1 -> Complex to Real-Imag/1
  imag/1 -> Real-Imag to Complex/2
  real/1 -> Real-Imag to Complex/1

== system Feeder_1/SM_NG/Single-Phase Dynamic Load34/model/PLL ==
  v (pu) : Inport
  freq (pu) : Inport  Port=2
  Gain : Gain  Gain=2*pi
  Gain1 : Gain  Gain=500
  Gain2 : Gain  Gain=freq
  IC : InitialCondition
  Integrator : Integrator
  Integrator1 : Integrator
  Product : Product  Inputs=**  RndMeth=Zero
  Sum1 : Sum  SaturateOnIntegerOverflow=on  InputSameDT=on  OutDataTypeStr=Inherit: Same as first input
  Trigonometric Function : Trigonometry  Operator=cos
  adaptive filter : Subsystem
  adaptive mean : Subsystem
  alpha (rad) : Outport
  wt : Outport  Port=2
  wires:
  freq (pu)/1 -> Gain2/1
  Gain2/1 -> adaptive filter/2(freq (Hz)), adaptive mean/2(freq (Hz)), Gain/1
  Trigonometric Function/1 -> Product/2
  adaptive mean/1(y) -> alpha (rad)/1
  Integrator1/1 -> Gain1/1
  Gain1/1 -> Sum1/1, adaptive mean/1(u)
  Sum1/1 -> Trigonometric Function/1
  Integrator/1 -> Sum1/2, wt/1
  Gain/1 -> Integrator/1
  adaptive filter/1(y) -> Integrator1/1
  Product/1 -> adaptive filter/1(u)
  v (pu)/1 -> IC/1
  IC/1 -> Product/1

== system Feeder_1/SM_NG/Single-Phase Dynamic Load34/model/Positive Sequence  current ==
  note: I1= (S/V1)'
  V1(pu) : Inport
  S_ext : Inport  Port=2
  Conj1 : Math  Operator=conj  SaturateOnIntegerOverflow=on
  Product : Product  Inputs=/*  SaturateOnIntegerOverflow=on  InputSameDT=on  OutDataTypeStr=Inherit: Same as first input
  pu>V : Gain  Gain=Vnom/sqrt(2)  SaturateOnIntegerOverflow=on  OutDataTypeStr=Inherit: Same as input  ParamDataTypeStr=Inherit: Same as input
  I1(A) : Outport
  wires:
  V1(pu)/1 -> pu>V/1
  Product/1 -> Conj1/1
  Conj1/1 -> I1(A)/1
  S_ext/1 -> Product/2
  pu>V/1 -> Product/1

== system Feeder_1/SM_NG/Single-Phase Dynamic Load35/model/Break  Alg. Loop ==
  In : Inport
  Complex to Real-Imag : ComplexToRealImag
  Real-Imag to Complex : RealImagToComplex
  imag : simulink_extras/Additional Linear/Transfer Fcn (with initial outputs)  N=[1]  D="[1000e-6  1]"  Y0=imag(I1_init*exp(-j*Pha_V0*pi/180))  U0=imag(I1_init*exp(-j*Pha_V0*pi/180))
  real : simulink_extras/Additional Linear/Transfer Fcn (with initial outputs)  N=[1]  D="[1000e-6  1]"  Y0=real(I1_init*exp(-j*Pha_V0*pi/180))  U0=real(I1_init*exp(-j*Pha_V0*pi/180))
  Out : Outport
  wires:
  imag/1 -> Real-Imag to Complex/2
  Complex to Real-Imag/2 -> imag/1
  real/1 -> Real-Imag to Complex/1
  Complex to Real-Imag/1 -> real/1
  Real-Imag to Complex/1 -> Out/1
  In/1 -> Complex to Real-Imag/1

== system Feeder_1/SM_NG/Single-Phase Dynamic Load35/model/PLL ==
  v (pu) : Inport
  freq (pu) : Inport  Port=2
  Gain : Gain  Gain=2*pi
  Gain1 : Gain  Gain=500
  Gain2 : Gain  Gain=freq
  IC : InitialCondition
  Integrator : Integrator
  Integrator1 : Integrator
  Product : Product  Inputs=**  RndMeth=Zero
  Sum1 : Sum  SaturateOnIntegerOverflow=on  InputSameDT=on  OutDataTypeStr=Inherit: Same as first input
  Trigonometric Function : Trigonometry  Operator=cos
  adaptive filter : Subsystem
  adaptive mean : Subsystem
  alpha (rad) : Outport
  wt : Outport  Port=2
  wires:
  freq (pu)/1 -> Gain2/1
  Gain2/1 -> adaptive filter/2(freq (Hz)), adaptive mean/2(freq (Hz)), Gain/1
  Trigonometric Function/1 -> Product/2
  adaptive mean/1(y) -> alpha (rad)/1
  Integrator1/1 -> Gain1/1
  Gain1/1 -> Sum1/1, adaptive mean/1(u)
  Sum1/1 -> Trigonometric Function/1
  Integrator/1 -> Sum1/2, wt/1
  Gain/1 -> Integrator/1
  adaptive filter/1(y) -> Integrator1/1
  Product/1 -> adaptive filter/1(u)
  v (pu)/1 -> IC/1
  IC/1 -> Product/1

== system Feeder_1/SM_NG/Single-Phase Dynamic Load35/model/Positive Sequence  current ==
  note: I1= (S/V1)'
  V1(pu) : Inport
  S_ext : Inport  Port=2
  Conj1 : Math  Operator=conj  SaturateOnIntegerOverflow=on
  Product : Product  Inputs=/*  SaturateOnIntegerOverflow=on  InputSameDT=on  OutDataTypeStr=Inherit: Same as first input
  pu>V : Gain  Gain=Vnom/sqrt(2)  SaturateOnIntegerOverflow=on  OutDataTypeStr=Inherit: Same as input  ParamDataTypeStr=Inherit: Same as input
  I1(A) : Outport
  wires:
  V1(pu)/1 -> pu>V/1
  Product/1 -> Conj1/1
  Conj1/1 -> I1(A)/1
  S_ext/1 -> Product/2
  pu>V/1 -> Product/1

== system Feeder_1/SM_NG/Single-Phase Dynamic Load36/model/Break  Alg. Loop1 ==
  In : Inport
  Complex to Real-Imag : ComplexToRealImag
  Real-Imag to Complex : RealImagToComplex
  imag : simulink_extras/Additional Linear/Transfer Fcn (with initial outputs)  N=[1]  D="[100e-6  1]"  Y0=imag(I1_init*exp(-j*Pha_V0*pi/180))  U0=imag(I1_init*exp(-j*Pha_V0*pi/180))
  real : simulink_extras/Additional Linear/Transfer Fcn (with initial outputs)  N=[1]  D="[100e-6  1]"  Y0=real(I1_init*exp(-j*Pha_V0*pi/180))  U0=real(I1_init*exp(-j*Pha_V0*pi/180))
  Out : Outport
  wires:
  Complex to Real-Imag/2 -> imag/1
  Complex to Real-Imag/1 -> real/1
  Real-Imag to Complex/1 -> Out/1
  In/1 -> Complex to Real-Imag/1
  imag/1 -> Real-Imag to Complex/2
  real/1 -> Real-Imag to Complex/1

== system Feeder_1/SM_NG/Single-Phase Dynamic Load36/model/PLL ==
  v (pu) : Inport
  freq (pu) : Inport  Port=2
  Gain : Gain  Gain=2*pi
  Gain1 : Gain  Gain=500
  Gain2 : Gain  Gain=freq
  IC : InitialCondition
  Integrator : Integrator
  Integrator1 : Integrator
  Product : Product  Inputs=**  RndMeth=Zero
  Sum1 : Sum  SaturateOnIntegerOverflow=on  InputSameDT=on  OutDataTypeStr=Inherit: Same as first input
  Trigonometric Function : Trigonometry  Operator=cos
  adaptive filter : Subsystem
  adaptive mean : Subsystem
  alpha (rad) : Outport
  wt : Outport  Port=2
  wires:
  freq (pu)/1 -> Gain2/1
  Gain2/1 -> adaptive filter/2(freq (Hz)), adaptive mean/2(freq (Hz)), Gain/1
  Trigonometric Function/1 -> Product/2
  adaptive mean/1(y) -> alpha (rad)/1
  Integrator1/1 -> Gain1/1
  Gain1/1 -> Sum1/1, adaptive mean/1(u)
  Sum1/1 -> Trigonometric Function/1
  Integrator/1 -> Sum1/2, wt/1
  Gain/1 -> Integrator/1
  adaptive filter/1(y) -> Integrator1/1
  Product/1 -> adaptive filter/1(u)
  v (pu)/1 -> IC/1
  IC/1 -> Product/1

== system Feeder_1/SM_NG/Single-Phase Dynamic Load36/model/Positive Sequence  current ==
  note: I1= (S/V1)'
  V1(pu) : Inport
  S_ext : Inport  Port=2
  Conj1 : Math  Operator=conj  SaturateOnIntegerOverflow=on
  Product : Product  Inputs=/*  SaturateOnIntegerOverflow=on  InputSameDT=on  OutDataTypeStr=Inherit: Same as first input
  pu>V : Gain  Gain=Vnom/sqrt(2)  SaturateOnIntegerOverflow=on  OutDataTypeStr=Inherit: Same as input  ParamDataTypeStr=Inherit: Same as input
  I1(A) : Outport
  wires:
  V1(pu)/1 -> pu>V/1
  Product/1 -> Conj1/1
  Conj1/1 -> I1(A)/1
  S_ext/1 -> Product/2
  pu>V/1 -> Product/1

== system Feeder_1/SM_NG/Single-Phase Dynamic Load37/model/Break  Alg. Loop1 ==
  In : Inport
  Complex to Real-Imag : ComplexToRealImag
  Real-Imag to Complex : RealImagToComplex
  imag : simulink_extras/Additional Linear/Transfer Fcn (with initial outputs)  N=[1]  D="[100e-6  1]"  Y0=imag(I1_init*exp(-j*Pha_V0*pi/180))  U0=imag(I1_init*exp(-j*Pha_V0*pi/180))
  real : simulink_extras/Additional Linear/Transfer Fcn (with initial outputs)  N=[1]  D="[100e-6  1]"  Y0=real(I1_init*exp(-j*Pha_V0*pi/180))  U0=real(I1_init*exp(-j*Pha_V0*pi/180))
  Out : Outport
  wires:
  Complex to Real-Imag/2 -> imag/1
  Complex to Real-Imag/1 -> real/1
  Real-Imag to Complex/1 -> Out/1
  In/1 -> Complex to Real-Imag/1
  imag/1 -> Real-Imag to Complex/2
  real/1 -> Real-Imag to Complex/1

== system Feeder_1/SM_NG/Single-Phase Dynamic Load37/model/PLL ==
  v (pu) : Inport
  freq (pu) : Inport  Port=2
  Gain : Gain  Gain=2*pi
  Gain1 : Gain  Gain=500
  Gain2 : Gain  Gain=freq
  IC : InitialCondition
  Integrator : Integrator
  Integrator1 : Integrator
  Product : Product  Inputs=**  RndMeth=Zero
  Sum1 : Sum  SaturateOnIntegerOverflow=on  InputSameDT=on  OutDataTypeStr=Inherit: Same as first input
  Trigonometric Function : Trigonometry  Operator=cos
  adaptive filter : Subsystem
  adaptive mean : Subsystem
  alpha (rad) : Outport
  wt : Outport  Port=2
  wires:
  freq (pu)/1 -> Gain2/1
  Gain2/1 -> adaptive filter/2(freq (Hz)), adaptive mean/2(freq (Hz)), Gain/1
  Trigonometric Function/1 -> Product/2
  adaptive mean/1(y) -> alpha (rad)/1
  Integrator1/1 -> Gain1/1
  Gain1/1 -> Sum1/1, adaptive mean/1(u)
  Sum1/1 -> Trigonometric Function/1
  Integrator/1 -> Sum1/2, wt/1
  Gain/1 -> Integrator/1
  adaptive filter/1(y) -> Integrator1/1
  Product/1 -> adaptive filter/1(u)
  v (pu)/1 -> IC/1
  IC/1 -> Product/1

== system Feeder_1/SM_NG/Single-Phase Dynamic Load37/model/Positive Sequence  current ==
  note: I1= (S/V1)'
  V1(pu) : Inport
  S_ext : Inport  Port=2
  Conj1 : Math  Operator=conj  SaturateOnIntegerOverflow=on
  Product : Product  Inputs=/*  SaturateOnIntegerOverflow=on  InputSameDT=on  OutDataTypeStr=Inherit: Same as first input
  pu>V : Gain  Gain=Vnom/sqrt(2)  SaturateOnIntegerOverflow=on  OutDataTypeStr=Inherit: Same as input  ParamDataTypeStr=Inherit: Same as input
  I1(A) : Outport
  wires:
  V1(pu)/1 -> pu>V/1
  Product/1 -> Conj1/1
  Conj1/1 -> I1(A)/1
  S_ext/1 -> Product/2
  pu>V/1 -> Product/1

== system Feeder_1/SM_NG/Single-Phase Dynamic Load38/model/Break  Alg. Loop1 ==
  In : Inport
  Complex to Real-Imag : ComplexToRealImag
  Real-Imag to Complex : RealImagToComplex
  imag : simulink_extras/Additional Linear/Transfer Fcn (with initial outputs)  N=[1]  D="[100e-6  1]"  Y0=imag(I1_init*exp(-j*Pha_V0*pi/180))  U0=imag(I1_init*exp(-j*Pha_V0*pi/180))
  real : simulink_extras/Additional Linear/Transfer Fcn (with initial outputs)  N=[1]  D="[100e-6  1]"  Y0=real(I1_init*exp(-j*Pha_V0*pi/180))  U0=real(I1_init*exp(-j*Pha_V0*pi/180))
  Out : Outport
  wires:
  Complex to Real-Imag/2 -> imag/1
  Complex to Real-Imag/1 -> real/1
  Real-Imag to Complex/1 -> Out/1
  In/1 -> Complex to Real-Imag/1
  imag/1 -> Real-Imag to Complex/2
  real/1 -> Real-Imag to Complex/1

== system Feeder_1/SM_NG/Single-Phase Dynamic Load38/model/PLL ==
  v (pu) : Inport
  freq (pu) : Inport  Port=2
  Gain : Gain  Gain=2*pi
  Gain1 : Gain  Gain=500
  Gain2 : Gain  Gain=freq
  IC : InitialCondition
  Integrator : Integrator
  Integrator1 : Integrator
  Product : Product  Inputs=**  RndMeth=Zero
  Sum1 : Sum  SaturateOnIntegerOverflow=on  InputSameDT=on  OutDataTypeStr=Inherit: Same as first input
  Trigonometric Function : Trigonometry  Operator=cos
  adaptive filter : Subsystem
  adaptive mean : Subsystem
  alpha (rad) : Outport
  wt : Outport  Port=2
  wires:
  freq (pu)/1 -> Gain2/1
  Gain2/1 -> adaptive filter/2(freq (Hz)), adaptive mean/2(freq (Hz)), Gain/1
  Trigonometric Function/1 -> Product/2
  adaptive mean/1(y) -> alpha (rad)/1
  Integrator1/1 -> Gain1/1
  Gain1/1 -> Sum1/1, adaptive mean/1(u)
  Sum1/1 -> Trigonometric Function/1
  Integrator/1 -> Sum1/2, wt/1
  Gain/1 -> Integrator/1
  adaptive filter/1(y) -> Integrator1/1
  Product/1 -> adaptive filter/1(u)
  v (pu)/1 -> IC/1
  IC/1 -> Product/1

== system Feeder_1/SM_NG/Single-Phase Dynamic Load38/model/Positive Sequence  current ==
  note: I1= (S/V1)'
  V1(pu) : Inport
  S_ext : Inport  Port=2
  Conj1 : Math  Operator=conj  SaturateOnIntegerOverflow=on
  Product : Product  Inputs=/*  SaturateOnIntegerOverflow=on  InputSameDT=on  OutDataTypeStr=Inherit: Same as first input
  pu>V : Gain  Gain=Vnom/sqrt(2)  SaturateOnIntegerOverflow=on  OutDataTypeStr=Inherit: Same as input  ParamDataTypeStr=Inherit: Same as input
  I1(A) : Outport
  wires:
  V1(pu)/1 -> pu>V/1
  Product/1 -> Conj1/1
  Conj1/1 -> I1(A)/1
  S_ext/1 -> Product/2
  pu>V/1 -> Product/1

== system Feeder_1/SM_NG/Single-Phase Dynamic Load39/model/Break  Alg. Loop1 ==
  In : Inport
  Complex to Real-Imag : ComplexToRealImag
  Real-Imag to Complex : RealImagToComplex
  imag : simulink_extras/Additional Linear/Transfer Fcn (with initial outputs)  N=[1]  D="[100e-6  1]"  Y0=imag(I1_init*exp(-j*Pha_V0*pi/180))  U0=imag(I1_init*exp(-j*Pha_V0*pi/180))
  real : simulink_extras/Additional Linear/Transfer Fcn (with initial outputs)  N=[1]  D="[100e-6  1]"  Y0=real(I1_init*exp(-j*Pha_V0*pi/180))  U0=real(I1_init*exp(-j*Pha_V0*pi/180))
  Out : Outport
  wires:
  Complex to Real-Imag/2 -> imag/1
  Complex to Real-Imag/1 -> real/1
  Real-Imag to Complex/1 -> Out/1
  In/1 -> Complex to Real-Imag/1
  imag/1 -> Real-Imag to Complex/2
  real/1 -> Real-Imag to Complex/1

== system Feeder_1/SM_NG/Single-Phase Dynamic Load39/model/PLL ==
  v (pu) : Inport
  freq (pu) : Inport  Port=2
  Gain : Gain  Gain=2*pi
  Gain1 : Gain  Gain=500
  Gain2 : Gain  Gain=freq
  IC : InitialCondition
  Integrator : Integrator
  Integrator1 : Integrator
  Product : Product  Inputs=**  RndMeth=Zero
  Sum1 : Sum  SaturateOnIntegerOverflow=on  InputSameDT=on  OutDataTypeStr=Inherit: Same as first input
  Trigonometric Function : Trigonometry  Operator=cos
  adaptive filter : Subsystem
  adaptive mean : Subsystem
  alpha (rad) : Outport
  wt : Outport  Port=2
  wires:
  freq (pu)/1 -> Gain2/1
  Gain2/1 -> adaptive filter/2(freq (Hz)), adaptive mean/2(freq (Hz)), Gain/1
  Trigonometric Function/1 -> Product/2
  adaptive mean/1(y) -> alpha (rad)/1
  Integrator1/1 -> Gain1/1
  Gain1/1 -> Sum1/1, adaptive mean/1(u)
  Sum1/1 -> Trigonometric Function/1
  Integrator/1 -> Sum1/2, wt/1
  Gain/1 -> Integrator/1
  adaptive filter/1(y) -> Integrator1/1
  Product/1 -> adaptive filter/1(u)
  v (pu)/1 -> IC/1
  IC/1 -> Product/1

== system Feeder_1/SM_NG/Single-Phase Dynamic Load39/model/Positive Sequence  current ==
  note: I1= (S/V1)'
  V1(pu) : Inport
  S_ext : Inport  Port=2
  Conj1 : Math  Operator=conj  SaturateOnIntegerOverflow=on
  Product : Product  Inputs=/*  SaturateOnIntegerOverflow=on  InputSameDT=on  OutDataTypeStr=Inherit: Same as first input
  pu>V : Gain  Gain=Vnom/sqrt(2)  SaturateOnIntegerOverflow=on  OutDataTypeStr=Inherit: Same as input  ParamDataTypeStr=Inherit: Same as input
  I1(A) : Outport
  wires:
  V1(pu)/1 -> pu>V/1
  Product/1 -> Conj1/1
  Conj1/1 -> I1(A)/1
  S_ext/1 -> Product/2
  pu>V/1 -> Product/1

== system Feeder_1/SM_NG/Single-Phase Dynamic Load40/model/Break  Alg. Loop1 ==
  In : Inport
  Complex to Real-Imag : ComplexToRealImag
  Real-Imag to Complex : RealImagToComplex
  imag : simulink_extras/Additional Linear/Transfer Fcn (with initial outputs)  N=[1]  D="[100e-6  1]"  Y0=imag(I1_init*exp(-j*Pha_V0*pi/180))  U0=imag(I1_init*exp(-j*Pha_V0*pi/180))
  real : simulink_extras/Additional Linear/Transfer Fcn (with initial outputs)  N=[1]  D="[100e-6  1]"  Y0=real(I1_init*exp(-j*Pha_V0*pi/180))  U0=real(I1_init*exp(-j*Pha_V0*pi/180))
  Out : Outport
  wires:
  Complex to Real-Imag/2 -> imag/1
  Complex to Real-Imag/1 -> real/1
  Real-Imag to Complex/1 -> Out/1
  In/1 -> Complex to Real-Imag/1
  imag/1 -> Real-Imag to Complex/2
  real/1 -> Real-Imag to Complex/1

== system Feeder_1/SM_NG/Single-Phase Dynamic Load40/model/PLL ==
  v (pu) : Inport
  freq (pu) : Inport  Port=2
  Gain : Gain  Gain=2*pi
  Gain1 : Gain  Gain=500
  Gain2 : Gain  Gain=freq
  IC : InitialCondition
  Integrator : Integrator
  Integrator1 : Integrator
  Product : Product  Inputs=**  RndMeth=Zero
  Sum1 : Sum  SaturateOnIntegerOverflow=on  InputSameDT=on  OutDataTypeStr=Inherit: Same as first input
  Trigonometric Function : Trigonometry  Operator=cos
  adaptive filter : Subsystem
  adaptive mean : Subsystem
  alpha (rad) : Outport
  wt : Outport  Port=2
  wires:
  freq (pu)/1 -> Gain2/1
  Gain2/1 -> adaptive filter/2(freq (Hz)), adaptive mean/2(freq (Hz)), Gain/1
  Trigonometric Function/1 -> Product/2
  adaptive mean/1(y) -> alpha (rad)/1
  Integrator1/1 -> Gain1/1
  Gain1/1 -> Sum1/1, adaptive mean/1(u)
  Sum1/1 -> Trigonometric Function/1
  Integrator/1 -> Sum1/2, wt/1
  Gain/1 -> Integrator/1
  adaptive filter/1(y) -> Integrator1/1
  Product/1 -> adaptive filter/1(u)
  v (pu)/1 -> IC/1
  IC/1 -> Product/1

== system Feeder_1/SM_NG/Single-Phase Dynamic Load40/model/Positive Sequence  current ==
  note: I1= (S/V1)'
  V1(pu) : Inport
  S_ext : Inport  Port=2
  Conj1 : Math  Operator=conj  SaturateOnIntegerOverflow=on
  Product : Product  Inputs=/*  SaturateOnIntegerOverflow=on  InputSameDT=on  OutDataTypeStr=Inherit: Same as first input
  pu>V : Gain  Gain=Vnom/sqrt(2)  SaturateOnIntegerOverflow=on  OutDataTypeStr=Inherit: Same as input  ParamDataTypeStr=Inherit: Same as input
  I1(A) : Outport
  wires:
  V1(pu)/1 -> pu>V/1
  Product/1 -> Conj1/1
  Conj1/1 -> I1(A)/1
  S_ext/1 -> Product/2
  pu>V/1 -> Product/1
